simulink model "MGBR"  (R2020a)
settings: Solver=VariableStepAuto  StartTime=0.0  StopTime=12  RelTol=1e-3
values from neighbouring files (symbols this model uses):
  g = 32.18    [MGU_K_Params.mat]
  m = 50    [MGU_K_Params.mat]
  R = 1.25    [MGU_K_Params.mat]
  v0 = 88    [MGU_K_Params.mat]
libraries: autolibshared x2, autolibcoupling x1, autolibsharedmappedengines x1, aerolibconvert2 x1
(part 3 of 3)

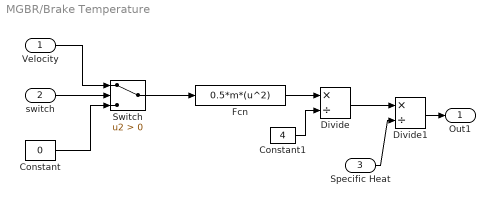
== system MGBR/Brake Temperature ==
  Velocity : Inport
  switch : Inport  Port=2
  Specific Heat : Inport  Port=3
  Constant : Constant  Value=0
  Constant1 : Constant  Value=4
  Divide : Product  Inputs=*/
  Divide1 : Product  Inputs=*/
  Fcn : Fcn  Expr=0.5*m*(u^2)
  Switch : Switch  Criteria=u2 > Threshold
  Out1 : Outport
  wires:
  Constant1/1 -> Divide/2
  Fcn/1 -> Divide/1
  Divide/1 -> Divide1/1
  Divide1/1 -> Out1/1
  Specific Heat/1 -> Divide1/2
  Constant/1 -> Switch/3
  Switch/1 -> Fcn/1
  Velocity/1 -> Switch/1
  switch/1 -> Switch/2

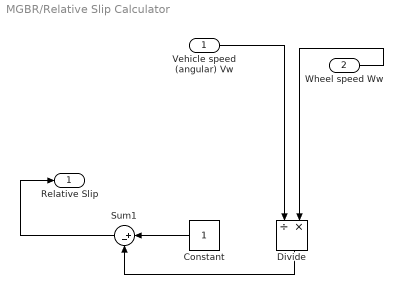
== system MGBR/Relative Slip Calculator ==
  Vehicle speed (angular) Vw : Inport
  Wheel speed Ww : Inport  Port=2
  Constant : Constant
  Divide : Product  Inputs=/*
  Sum1 : Sum  Inputs=|+-
  Relative Slip : Outport  VectorParamsAs1DForOutWhenUnconnected=off
  wires:
  Divide/1 -> Sum1/2
  Sum1/1 -> Relative Slip/1
  Constant/1 -> Sum1/1
  Wheel speed Ww/1 -> Divide/2
  Vehicle speed (angular) Vw/1 -> Divide/1
